simulink model "LookupTableND"  (R2017b)
settings: Solver=FixedStepDiscrete  StartTime=0.0  StopTime=10.0  FixedStep=0.200000  RelTol=1e-3  EnableMultiTasking=on
settings Model: Creator=hbourbou  LastModifiedBy=hbourbou
settings DataIOCC: LimitDataPoints=on  SaveFormat=StructureWithTime
settings OptimizationCC: LifeSpan=inf
settings DebuggingCC: SFUnexpectedBacktrackingDiag=warning  SFNoUnconditionalDefaultTransitionDiag=warning  SFExecutionAtInitializationDiag=none
settings HardwareCC: ProdBitPerSizeT=32  ProdBitPerPtrDiffT=32  ProdWordSize=32  ProdHWDeviceType=Specified
settings ModelReferenceCC: PropagateSignalLabelsOutOfModel=off
settings CodeAppCC: StateflowObjectComments=on
settings GRTTargetCC: TargetLangStandard=C89/C90 (ANSI)
settings ConfigComp: CovMetricSettings=dw  CovHtmlReporting=on  CovSaveCumulativeToWorkspaceVar=on  CovSaveSingleToWorkspaceVar=on  CovExternalEMLEnable=off

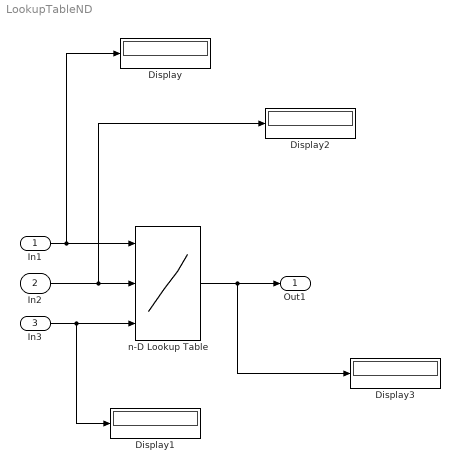
== system LookupTableND ==
  In1 : Inport
  In2 : Inport  Port=2
  In3 : Inport  Port=3
  Display{,1..3} (4 alike) : Display
  n-D Lookup Table : Lookup_n-D  NumberOfTableDimensions=3  BreakpointsForDimension3=[5, 7]  Table=reshape(repmat([4 5 6;16 19 20;10 18 23],1,2),[3,3,2])  InternalRulePriority=Speed  RndMeth=Simplest  InputSameDT=on
  Out1 : Outport
  wires:
  In1/1 -> Display/1, n-D Lookup Table/1
  In2/1 -> Display2/1, n-D Lookup Table/2
  In3/1 -> Display1/1, n-D Lookup Table/3
  n-D Lookup Table/1 -> Display3/1, Out1/1
